simulink model "Control_R2016a"  (R2016a)
settings: Solver=ode4  SolverMode=SingleTasking  StartTime=0  StopTime=1000  FixedStep=ConfParam.confOrbit.dt  RelTol=1e-3
undefined symbols (not defined in the file): ConfParam
libraries: Command x1, Date x1, KepOrbit x1, Estimator x1, BdotController x1, IGRF x1, SunEphemeris_MathWorks x1, MTB x1, Magnetometer x1, AeroTorqueA x1, ChangeFrame x1, Qinverse x1
settings Model: Creator=Cédric  LastModifiedBy=Cédric
settings DataIOCC: SaveTime=off
settings DebuggingCC: MultiTaskRateTransMsg=warning  SFUnexpectedBacktrackingDiag=error  SFNoUnconditionalDefaultTransitionDiag=error
settings GRTTargetCC: TargetLangStandard=C99 (ISO)  GeneratePreprocessorConditionals=Use local settings
settings ConfigComp: CovMetricSettings=dwe  CovHtmlReporting=off  CovSaveCumulativeToWorkspaceVar=off  CovSaveSingleToWorkspaceVar=off  CovExternalEMLEnable=on

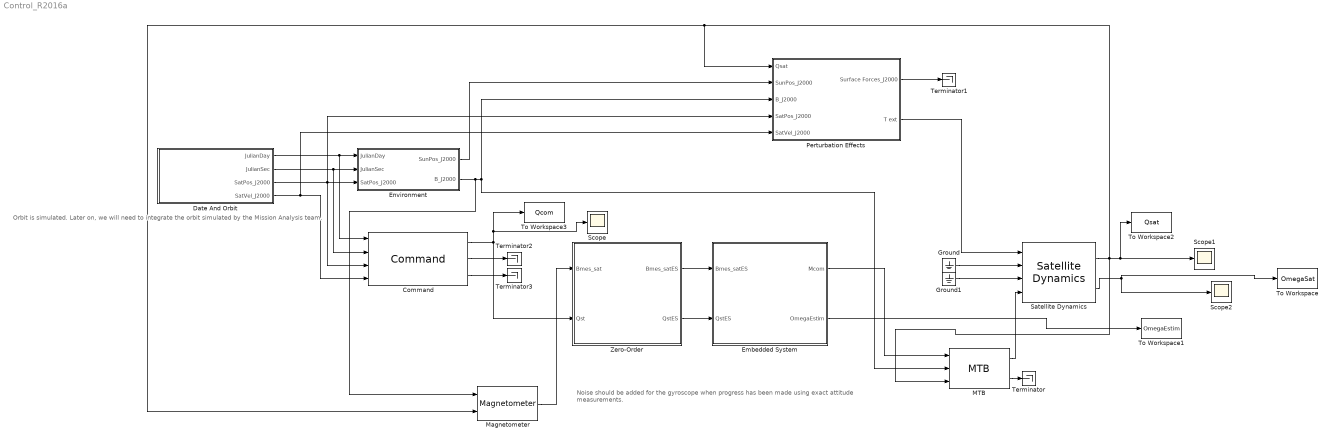
== system Control_R2016a ==
  note: Orbit is simulated. Later on, we will need to integrate the orbit simulated by the Mission Analysis team.
  note: Noise should be added for the gyroscope when progress has been made using exact attitude measurements.
  Command : Command/Command
  Date And Orbit : Subsystem
  Embedded System : Subsystem
  Environment : Subsystem
  Ground : Ground
  Ground1 : Ground
  MTB : MTB/MTB
  Magnetometer : Magnetometer/Magnetometer
  Perturbation Effects : Subsystem
  Satellite Dynamics : SatDyn/Satellite Dynamics
  Scope : Scope
  Scope1 : Scope
  Scope2 : Scope
  Terminator{,1..3} (4 alike) : Terminator
  To Workspace : ToWorkspace  VariableName=OmegaSat  SaveFormat=Timeseries  SampleTime=-1
  To Workspace1 : ToWorkspace  VariableName=OmegaEstim  SaveFormat=Timeseries  SampleTime=-1
  To Workspace2 : ToWorkspace  VariableName=Qsat  SaveFormat=Timeseries  SampleTime=-1
  To Workspace3 : ToWorkspace  VariableName=Qcom  SaveFormat=Timeseries  SampleTime=-1
  Zero-Order : Subsystem
  wires:
  Date And Orbit/1(JulianDay) -> Command/1, Environment/1(JulianDay)
  Date And Orbit/2(JulianSec) -> Command/2, Environment/2(JulianSec)
  Date And Orbit/3(SatPos_J2000) -> Perturbation Effects/4(SatPos_J2000), Command/3, Environment/3(SatPos_J2000)
  Environment/2(B_J2000) -> Magnetometer/1, MTB/2, Perturbation Effects/3(B_J2000)
  Date And Orbit/4(SatVel_J2000) -> Perturbation Effects/5(SatVel_J2000), Command/4
  Environment/1(SunPos_J2000) -> Perturbation Effects/2(SunPos_J2000)
  Zero-Order/1(Bmes_satES) -> Embedded System/1(Bmes_satES)
  Zero-Order/2(QstES) -> Embedded System/2(QstES)
  Embedded System/1(Mcom) -> MTB/1
  Perturbation Effects/2(T ext) -> Satellite Dynamics/1
  MTB/1 -> Satellite Dynamics/4
  Magnetometer/1 -> Zero-Order/1(Bmes_sat)
  Command/1 -> Scope/1, To Workspace3/1, Zero-Order/2(Qst)
  Satellite Dynamics/1 -> Scope1/1, To Workspace2/1, Perturbation Effects/1(Qsat), Magnetometer/2, MTB/3
  Ground/1 -> Satellite Dynamics/2
  Ground1/1 -> Satellite Dynamics/3
  MTB/2 -> Terminator/1
  Embedded System/2(OmegaEstim) -> To Workspace1/1
  Satellite Dynamics/2 -> Scope2/1, To Workspace/1
  Perturbation Effects/1(Surface Forces_J2000) -> Terminator1/1
  Command/3 -> Terminator3/1
  Command/2 -> Terminator2/1

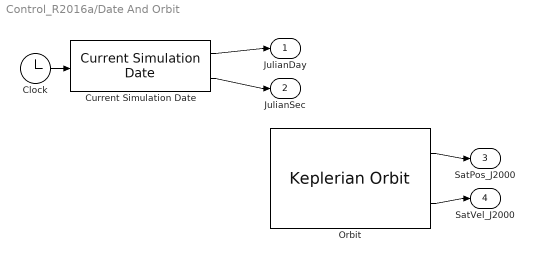
== system Control_R2016a/Date And Orbit ==
  Clock : Clock
  Current Simulation Date : Date/Current Simulation Date
  Orbit : KepOrbit/Keplerian Orbit
  JulianDay : Outport
  JulianSec : Outport  Port=2
  SatPos_J2000 : Outport  Port=3
  SatVel_J2000 : Outport  Port=4
  wires:
  Current Simulation Date/1 -> JulianDay/1
  Current Simulation Date/2 -> JulianSec/1
  Clock/1 -> Current Simulation Date/1
  Orbit/1 -> SatPos_J2000/1
  Orbit/2 -> SatVel_J2000/1

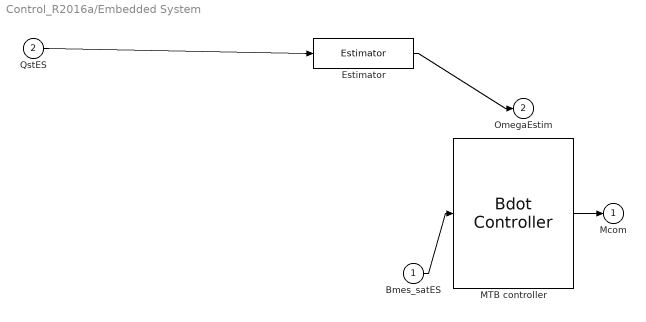
== system Control_R2016a/Embedded System ==
  Bmes_satES : Inport
  QstES : Inport  Port=2
  Estimator : Estimator/Estimator
  MTB controller : BdotController/Bdot Controller
  Mcom : Outport
  OmegaEstim : Outport  Port=2
  wires:
  QstES/1 -> Estimator/1
  Estimator/1 -> OmegaEstim/1
  Bmes_satES/1 -> MTB controller/1
  MTB controller/1 -> Mcom/1

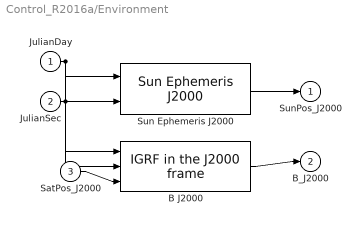
== system Control_R2016a/Environment ==
  JulianDay : Inport
  JulianSec : Inport  Port=2
  SatPos_J2000 : Inport  Port=3
  B J2000 : IGRF/IGRF in the J2000 frame
  Sun Ephemeris J2000 : SunEphemeris_MathWorks/Sun Ephemeris J2000
  SunPos_J2000 : Outport
  B_J2000 : Outport  Port=2
  wires:
  Sun Ephemeris J2000/1 -> SunPos_J2000/1
  JulianDay/1 -> Sun Ephemeris J2000/1, B J2000/1
  JulianSec/1 -> Sun Ephemeris J2000/2, B J2000/2
  SatPos_J2000/1 -> B J2000/3
  B J2000/1 -> B_J2000/1

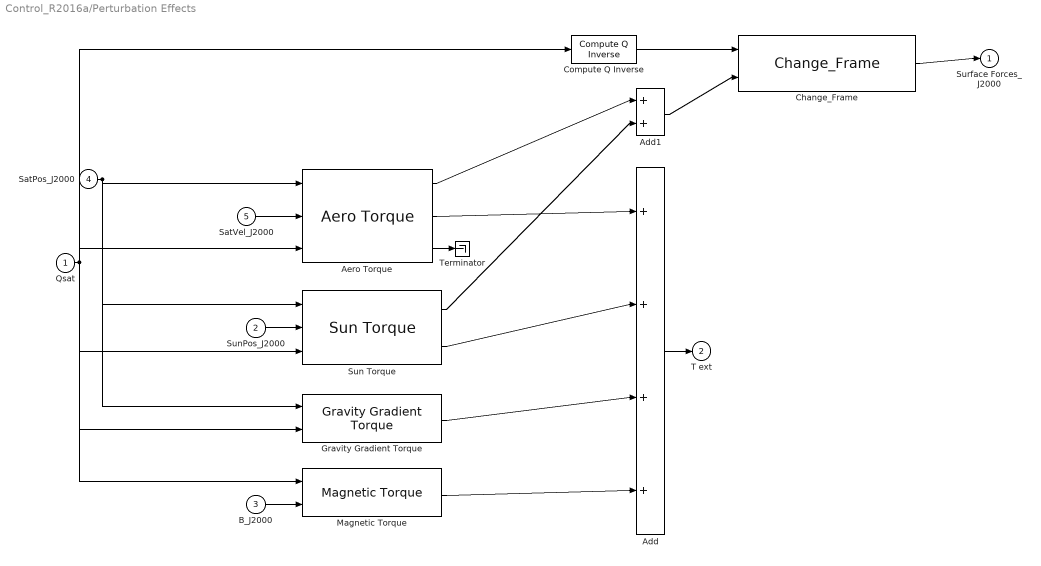
== system Control_R2016a/Perturbation Effects ==
  Qsat : Inport
  SunPos_J2000 : Inport  Port=2
  B_J2000 : Inport  Port=3
  SatPos_J2000 : Inport  Port=4
  SatVel_J2000 : Inport  Port=5
  Add : Sum  Inputs=++++
  Add1 : Sum
  Aero Torque : AeroTorqueA/Aero Torque
  Change_Frame : ChangeFrame/Change_Frame
  Compute Q Inverse : Qinverse/Compute Q Inverse
  Gravity Gradient Torque : GravGradTorque/Gravity Gradient Torque
  Magnetic Torque : MagnTorque/Magnetic Torque
  Sun Torque : SunTorqueA/Sun Torque
  Terminator : Terminator
  Surface Forces_J2000 : Outport
  T ext : Outport  Port=2
  wires:
  Compute Q Inverse/1 -> Change_Frame/1
  Change_Frame/1 -> Surface Forces_J2000/1
  Qsat/1 -> Compute Q Inverse/1, Gravity Gradient Torque/2, Sun Torque/3, Magnetic Torque/1, Aero Torque/3
  SunPos_J2000/1 -> Sun Torque/2
  B_J2000/1 -> Magnetic Torque/2
  SatPos_J2000/1 -> Sun Torque/1, Gravity Gradient Torque/1, Aero Torque/1
  SatVel_J2000/1 -> Aero Torque/2
  Aero Torque/3 -> Terminator/1
  Add1/1 -> Change_Frame/2
  Aero Torque/1 -> Add1/1
  Sun Torque/1 -> Add1/2
  Add/1 -> T ext/1
  Aero Torque/2 -> Add/1
  Sun Torque/2 -> Add/2
  Gravity Gradient Torque/1 -> Add/3
  Magnetic Torque/1 -> Add/4

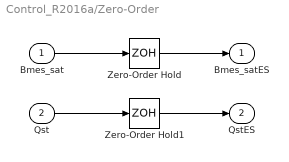
== system Control_R2016a/Zero-Order ==
  Bmes_sat : Inport
  Qst : Inport  Port=2
  Zero-Order Hold : ZeroOrderHold  SampleTime=1/ConfParam.confES.frequency
  Zero-Order Hold1 : ZeroOrderHold  SampleTime=1/ConfParam.confES.frequency
  Bmes_satES : Outport
  QstES : Outport  Port=2
  wires:
  Bmes_sat/1 -> Zero-Order Hold/1
  Zero-Order Hold/1 -> Bmes_satES/1
  Qst/1 -> Zero-Order Hold1/1
  Zero-Order Hold1/1 -> QstES/1
